simulink model "NucleoTesterScreen"  (R2018a)
settings: Solver=FixedStepAuto  StartTime=0.0  StopTime=10000  FixedStep=0.01  RelTol=1e-3
undefined symbols (not defined in the file): serial
libraries: instrumentlib x6
settings Model: Creator=SIMONE  LastModifiedBy=Salvatore

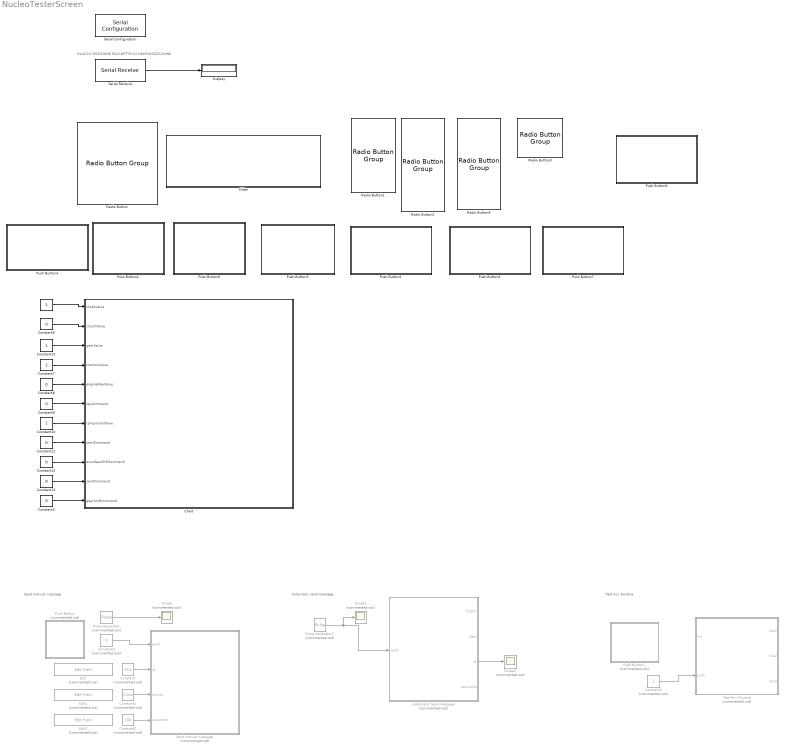
== system NucleoTesterScreen ==
  note: BLOCCO RICEZIONE PACCHETTO DI SINCRONIZZAZIONE
  note: Test Acc Routine
  note: Automatic send message
  note: Send manual message
  " " : Constant  OutDataTypeStr=uint8
  Automatic Send message : Stateflow chart  Commented=on  TreatAsAtomicUnit=on
  Chart : Stateflow chart  TreatAsAtomicUnit=on
  Constant : Constant  Commented=on  Value=513  OutDataTypeStr=uint16
  Constant1 : Constant  Commented=on  Value=21000  OutDataTypeStr=uint16
  Constant10 : Constant  OutDataTypeStr=uint8
  Constant{5,9,11..13} (5 alike) : Constant  Value=0  OutDataTypeStr=uint16
  Constant15 : Constant  OutDataTypeStr=uint8
  Constant2 : Constant  Commented=on  Value=100  OutDataTypeStr=uint16
  Constant3 : Constant  Commented=on  Value=0
  Constant4 : Constant  Commented=on
  Constant6 : Constant  Value=0  OutDataTypeStr=uint8
  Constant7 : Constant  Value=2  OutDataTypeStr=uint8
  Constant8 : Constant  Value=0  OutDataTypeStr=uint8
  Display : Display
  Edit : EditField  Commented=on  WebBlockId=20  LabelPosition=Hide  Alignment=Center
  Edit1 : EditField  Commented=on  WebBlockId=23  LabelPosition=Hide  Alignment=Center
  Edit2 : EditField  Commented=on  WebBlockId=25  LabelPosition=Hide  Alignment=Center
  Pulse Generator : DiscretePulseGenerator  Commented=on  PulseType=Time based  Period=10  PulseWidth=2%  PhaseDelay=1
  Pulse Generator1 : DiscretePulseGenerator  Commented=on  PulseType=Time based  Period=0.2  PulseWidth=25%  PhaseDelay=1
  Push Button : Subsystem  Commented=on  DialogController=hmiCreateDDGDialog  IsWebBlock=on  mask(MWDashboardBlock){webBlockId=12b47424-de0c-4dac-be92-db9266863398, webBlockType=pushbutton, ShowInLibBrwoser=on, ShowInitialText=on, HMISrcModelName=NucleoTesterScreen}
      mask prompts: webBlockId "WebBlock Id"; webBlockType "WebBlock Type"; HMISrcModelName "Source Model"
      mask help: SimulinkHMI:dialogs:PushButtonDialogDesc
      mask Help: helpview([docroot '/mapfiles/simulink.map'], 'hmi_push_button')
      mask Display:
      | model = bdroot(gcb);
      | if strcmp(get_param(model,'BlockDiagramType'), 'library')
      |     image([(matlabroot) '/toolbox/simulink/hmi/icons/PushButton.png']);
      | end
  Push Button1 : Subsystem  Commented=on  DialogController=hmiCreateDDGDialog  IsWebBlock=on  mask(MWDashboardBlock){webBlockId=b87c9129-2ae4-4d53-baa3-891c0a6e6068, webBlockType=pushbutton, ShowInLibBrwoser=on, ShowInitialText=on, HMISrcModelName=NucleoTesterScreen}
      mask prompts: webBlockId "WebBlock Id"; webBlockType "WebBlock Type"; HMISrcModelName "Source Model"
      mask help: SimulinkHMI:dialogs:PushButtonDialogDesc
      mask Help: helpview([docroot '/mapfiles/simulink.map'], 'hmi_push_button')
      mask Display:
      | model = bdroot(gcb);
      | if strcmp(get_param(model,'BlockDiagramType'), 'library')
      |     image([(matlabroot) '/toolbox/simulink/hmi/icons/PushButton.png']);
      | end
  Push Button2 : Subsystem  DialogController=hmiCreateDDGDialog  IsWebBlock=on  mask(MWDashboardBlock){webBlockId=bebfbbc1-03e8-40c0-bb91-fd2048b7631c, webBlockType=pushbutton, ShowInLibBrwoser=on, ShowInitialText=on, HMISrcModelName=NucleoTesterScreen}
      mask prompts: webBlockId "WebBlock Id"; webBlockType "WebBlock Type"; HMISrcModelName "Source Model"
      mask help: SimulinkHMI:dialogs:PushButtonDialogDesc
      mask Help: helpview([docroot '/mapfiles/simulink.map'], 'hmi_push_button')
      mask Display:
      | model = bdroot(gcb);
      | if strcmp(get_param(model,'BlockDiagramType'), 'library')
      |     image([(matlabroot) '/toolbox/simulink/hmi/icons/PushButton.png']);
      | end
  Push Button3 : Subsystem  DialogController=hmiCreateDDGDialog  IsWebBlock=on  mask(MWDashboardBlock){webBlockId=c39a8395-b875-430f-96b1-fe620fcd5c72, webBlockType=pushbutton, ShowInLibBrwoser=on, ShowInitialText=on, HMISrcModelName=NucleoTesterScreen}
      mask prompts: webBlockId "WebBlock Id"; webBlockType "WebBlock Type"; HMISrcModelName "Source Model"
      mask help: SimulinkHMI:dialogs:PushButtonDialogDesc
      mask Help: helpview([docroot '/mapfiles/simulink.map'], 'hmi_push_button')
      mask Display:
      | model = bdroot(gcb);
      | if strcmp(get_param(model,'BlockDiagramType'), 'library')
      |     image([(matlabroot) '/toolbox/simulink/hmi/icons/PushButton.png']);
      | end
  Push Button4 : Subsystem  DialogController=hmiCreateDDGDialog  IsWebBlock=on  mask(MWDashboardBlock){webBlockId=2fda76cb-15c6-45e5-b8fc-bd031a2f9463, webBlockType=pushbutton, ShowInLibBrwoser=on, ShowInitialText=on, HMISrcModelName=NucleoTesterScreen}
      mask prompts: webBlockId "WebBlock Id"; webBlockType "WebBlock Type"; HMISrcModelName "Source Model"
      mask help: SimulinkHMI:dialogs:PushButtonDialogDesc
      mask Help: helpview([docroot '/mapfiles/simulink.map'], 'hmi_push_button')
      mask Display:
      | model = bdroot(gcb);
      | if strcmp(get_param(model,'BlockDiagramType'), 'library')
      |     image([(matlabroot) '/toolbox/simulink/hmi/icons/PushButton.png']);
      | end
  Push Button5 : Subsystem  DialogController=hmiCreateDDGDialog  IsWebBlock=on  mask(MWDashboardBlock){webBlockId=fa35870d-30f4-4e57-b9ad-d2f6e23801ce, webBlockType=pushbutton, ShowInLibBrwoser=on, ShowInitialText=on, HMISrcModelName=NucleoTesterScreen}
      mask prompts: webBlockId "WebBlock Id"; webBlockType "WebBlock Type"; HMISrcModelName "Source Model"
      mask help: SimulinkHMI:dialogs:PushButtonDialogDesc
      mask Help: helpview([docroot '/mapfiles/simulink.map'], 'hmi_push_button')
      mask Display:
      | model = bdroot(gcb);
      | if strcmp(get_param(model,'BlockDiagramType'), 'library')
      |     image([(matlabroot) '/toolbox/simulink/hmi/icons/PushButton.png']);
      | end
  Push Button6 : Subsystem  DialogController=hmiCreateDDGDialog  IsWebBlock=on  mask(MWDashboardBlock){webBlockId=f57953b8-e9ec-4930-bf26-42a61eaad514, webBlockType=pushbutton, ShowInLibBrwoser=on, ShowInitialText=on, HMISrcModelName=NucleoTesterScreen}
      mask prompts: webBlockId "WebBlock Id"; webBlockType "WebBlock Type"; HMISrcModelName "Source Model"
      mask help: SimulinkHMI:dialogs:PushButtonDialogDesc
      mask Help: helpview([docroot '/mapfiles/simulink.map'], 'hmi_push_button')
      mask Display:
      | model = bdroot(gcb);
      | if strcmp(get_param(model,'BlockDiagramType'), 'library')
      |     image([(matlabroot) '/toolbox/simulink/hmi/icons/PushButton.png']);
      | end
  Push Button7 : Subsystem  DialogController=hmiCreateDDGDialog  IsWebBlock=on  mask(MWDashboardBlock){webBlockId=9216e8e9-0fef-4c72-b5a1-64b944c1ca6f, webBlockType=pushbutton, ShowInLibBrwoser=on, ShowInitialText=on, HMISrcModelName=NucleoTesterScreen}
      mask prompts: webBlockId "WebBlock Id"; webBlockType "WebBlock Type"; HMISrcModelName "Source Model"
      mask help: SimulinkHMI:dialogs:PushButtonDialogDesc
      mask Help: helpview([docroot '/mapfiles/simulink.map'], 'hmi_push_button')
      mask Display:
      | model = bdroot(gcb);
      | if strcmp(get_param(model,'BlockDiagramType'), 'library')
      |     image([(matlabroot) '/toolbox/simulink/hmi/icons/PushButton.png']);
      | end
  Push Button8 : Subsystem  DialogController=hmiCreateDDGDialog  IsWebBlock=on  mask(MWDashboardBlock){webBlockId=35ec2f2d-26a3-46c4-8c27-c0d592bab191, webBlockType=pushbutton, ShowInLibBrwoser=on, ShowInitialText=on, HMISrcModelName=NucleoTesterScreen}
      mask prompts: webBlockId "WebBlock Id"; webBlockType "WebBlock Type"; HMISrcModelName "Source Model"
      mask help: SimulinkHMI:dialogs:PushButtonDialogDesc
      mask Help: helpview([docroot '/mapfiles/simulink.map'], 'hmi_push_button')
      mask Display:
      | model = bdroot(gcb);
      | if strcmp(get_param(model,'BlockDiagramType'), 'library')
      |     image([(matlabroot) '/toolbox/simulink/hmi/icons/PushButton.png']);
      | end
  Push Button9 : Subsystem  DialogController=hmiCreateDDGDialog  IsWebBlock=on  mask(MWDashboardBlock){webBlockId=fbcfdafe-b282-4dbd-a33a-70d3112159dd, webBlockType=pushbutton, ShowInLibBrwoser=on, ShowInitialText=on, HMISrcModelName=NucleoTesterScreen}
      mask prompts: webBlockId "WebBlock Id"; webBlockType "WebBlock Type"; HMISrcModelName "Source Model"
      mask help: SimulinkHMI:dialogs:PushButtonDialogDesc
      mask Help: helpview([docroot '/mapfiles/simulink.map'], 'hmi_push_button')
      mask Display:
      | model = bdroot(gcb);
      | if strcmp(get_param(model,'BlockDiagramType'), 'library')
      |     image([(matlabroot) '/toolbox/simulink/hmi/icons/PushButton.png']);
      | end
  Radio Button : RadioButtonGroup  WebBlockId=105  SelectedLabel=Skidpad  ButtonGroupName=MODE
      settings: Values={{'Endurance', 'Acceleration', 'Autocross', 'Skidpad', 'Debug'}, [2 3 0 1 4]}
  Radio Button1 : RadioButtonGroup  WebBlockId=124  SelectedLabel=1  ButtonGroupName=GEAR
      settings: Values={{'1', 'N', '2', '3', '4', '5'}, [1 0 2 3 4 5]}
  Radio Button2 : RadioButtonGroup  WebBlockId=128  SelectedLabel=2  ButtonGroupName=TRACTION
      settings: Values={{'0', '1', '2', '3', '4', '5', '6', '7'}, [0 1 2 3 4 5 6 7]}
  Radio Button3 : RadioButtonGroup  WebBlockId=126  SelectedLabel=MAP 2  ButtonGroupName=ENGINE_MAP
      settings: Values={{'MAP 1', 'MAP 2'}, [1 2]}
  Radio Button4 : RadioButtonGroup  WebBlockId=127  SelectedLabel=1  ButtonGroupName=RPM_LIMITER
      settings: Values={{'0', '1', '2', '3', '4', '5', '6', '7'}, [0 1 2 3 4 5 6 7]}
  Scope : Scope  Commented=on
  Scope1 : Scope  Commented=on
  Scope2 : Scope  Commented=on
  Send manual message : Stateflow chart  Commented=on  TreatAsAtomicUnit=on
  Serial Configuration : instrumentlib/Serial Configuration  Priority=-200000  ComPortMenu=<Please select a port...>  ComPort=COM9  ObjConstructor=serial('COM9');  BaudRate=115200  DataBits=8  Parity=none  StopBits=1  FlowControl=none  Timeout=10  ByteOrder=LittleEndian
  Serial Receive : instrumentlib/Serial Receive  ComPortMenu=<Please select a port...>  ComPort=COM9  ObjConstructor=serial('COM9');  Terminator=<none>  DataSize="[1  1]"  DataType=uint8  EnableBlockingMode=on  ActionDataUnavailable=Output last received value  CustomValue=0  SampleTime=0.01
  Slider : Subsystem  DialogController=hmiCreateDDGDialog  IsWebBlock=on  mask(MWDashboardBlock){webBlockId=fe872d36-e610-44f7-a113-dcc518d376f0, webBlockType=slider, ShowInLibBrowser=on, ShowInitialText=on, HMISrcModelName=NucleoTesterScreen}
      mask prompts: webBlockId "WebBlock Id"; webBlockType "WebBlock Type"; HMISrcModelName "Source Model"
      mask help: SimulinkHMI:dialogs:SliderDialogDesc
      mask Help: helpview([docroot '/mapfiles/simulink.map'], 'hmi_slider')
      mask Display:
      | if strcmp(get_param(bdroot(gcb),'BlockDiagramType'), 'library')
      |     image([(matlabroot) '/toolbox/simulink/hmi/icons/Slider.png']);
      | end
  Test Acc Routine : Subsystem  Commented=on
  wires:
  Constant2/1 -> Send manual message/4(secondInt)
  Constant1/1 -> Send manual message/3(firstInt)
  Constant/1 -> Send manual message/2(id)
  Pulse Generator/1 -> Scope/1
  Pulse Generator1/1 -> Scope1/1, Automatic Send message/1(push)
  Automatic Send message/3(id) -> Scope2/1
  Constant3/1 -> Send manual message/1(push)
  Constant4/1 -> Test Acc Routine/2(push)
  Serial Receive/1 -> Display/1
  " "/1 -> Chart/1(modeValue)
  Constant6/1 -> Chart/2(clutchValue)
  Constant15/1 -> Chart/3(gearValue)
  Constant7/1 -> Chart/4(tractionValue)
  Constant8/1 -> Chart/5(engineMapValue)
  Constant9/1 -> Chart/6(keyCommand)
  Constant10/1 -> Chart/7(rpmLimiterValue)
  Constant11/1 -> Chart/8(startCommand)
  Constant12/1 -> Chart/9(autoGearShiftCommand)
  Constant13/1 -> Chart/10(sendCommand)
  Constant5/1 -> Chart/11(gearShiftCommand)

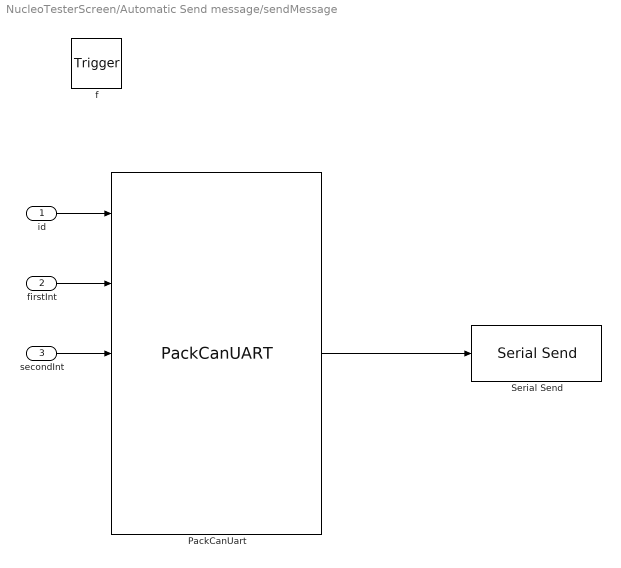
== system NucleoTesterScreen/Automatic Send message/sendMessage ==
  id : Inport  OutDataTypeStr=uint16  PortDimensions=1
  firstInt : Inport  Port=2  OutDataTypeStr=uint16  PortDimensions=1
  secondInt : Inport  Port=3  OutDataTypeStr=uint16  PortDimensions=1
  f : TriggerPort  TriggerType=function-call  VariantControl=(inherit)
      settings: CopyFcn=Stateflow.SLINSF.SimulinkMan.removeBlockPreDeleteFcn  PreDeleteFcn=Stateflow.SLINSF.SimulinkMan.unsafePredeleteFcn
  PackCanUart : S-Function  FunctionName=PackCanUART  SFunctionDeploymentMode=off  EnableBusSupport=off
  Serial Send : instrumentlib/Serial Send  ComPortMenu=<Please select a port...>  ComPort=COM4  ObjConstructor=serial('COM4');  Header=hdr  Terminator=<none>  EnableBlockingMode=on
  wires:
  secondInt/1 -> PackCanUart/3
  firstInt/1 -> PackCanUart/2
  PackCanUart/1 -> Serial Send/1
  id/1 -> PackCanUart/1

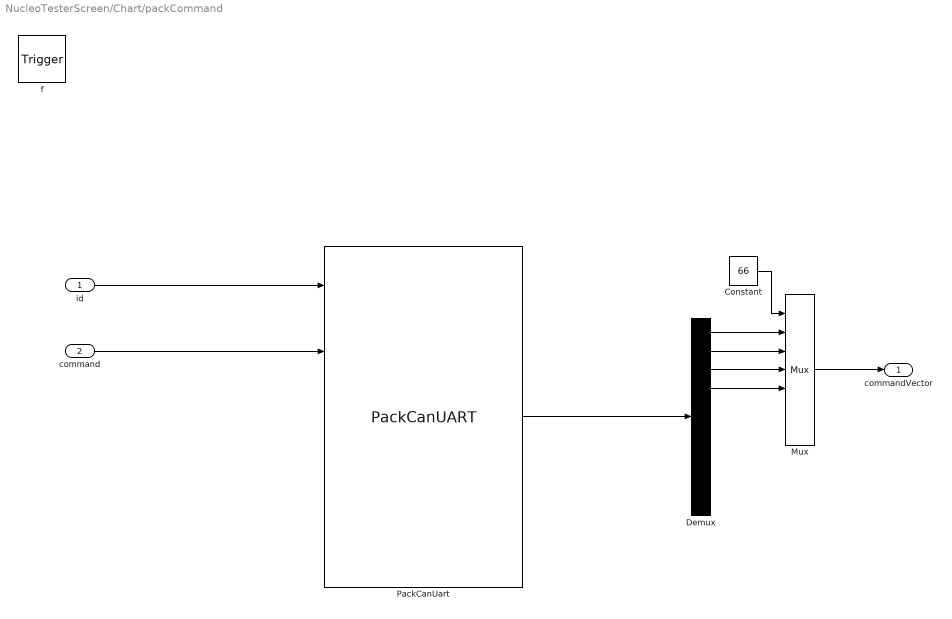
== system NucleoTesterScreen/Chart/packCommand ==
  id : Inport  OutDataTypeStr=uint16  PortDimensions=1
  command : Inport  Port=2  OutDataTypeStr=uint16  PortDimensions=1
  f : TriggerPort  TriggerType=function-call  VariantControl=(inherit)
      settings: CopyFcn=Stateflow.SLINSF.SimulinkMan.removeBlockPreDeleteFcn  PreDeleteFcn=Stateflow.SLINSF.SimulinkMan.unsafePredeleteFcn
  Constant : Constant  Value=66  OutDataTypeStr=uint8
  Demux : Demux  Outputs=10
  Mux : Mux  Inputs=7
  PackCanUart : S-Function  FunctionName=PackCanUART  SFunctionDeploymentMode=off  EnableBusSupport=off
  commandVector : Outport  PortDimensions=[1 7]
  wires:
  id/1 -> PackCanUart/1
  command/1 -> PackCanUart/2
  PackCanUart/1 -> Demux/1
  Mux/1 -> commandVector/1
  Demux/1 -> Mux/2
  Demux/2 -> Mux/3
  Demux/3 -> Mux/4
  Demux/4 -> Mux/5
  Constant/1 -> Mux/1

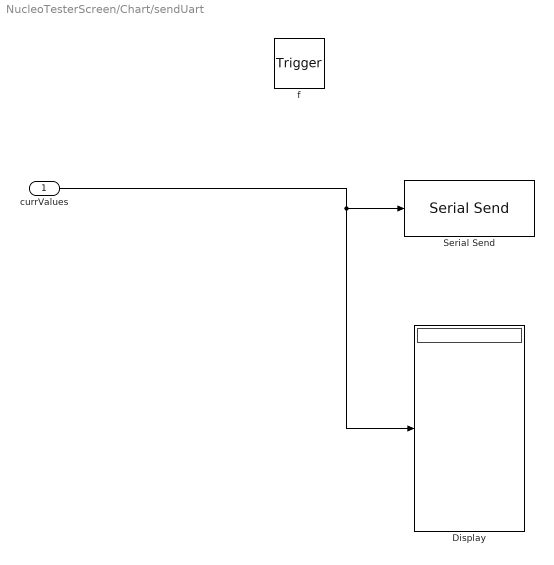
== system NucleoTesterScreen/Chart/sendUart ==
  currValues : Inport  OutDataTypeStr=uint8  PortDimensions=[1,7]
  f : TriggerPort  TriggerType=function-call  VariantControl=(inherit)
      settings: CopyFcn=Stateflow.SLINSF.SimulinkMan.removeBlockPreDeleteFcn  PreDeleteFcn=Stateflow.SLINSF.SimulinkMan.unsafePredeleteFcn
  Display : Display
  Serial Send : instrumentlib/Serial Send  ComPortMenu=COM9  ComPort=COM9  ObjConstructor=serial('COM9');  Terminator=<none>  EnableBlockingMode=on
  wires:
  currValues/1 -> Display/1, Serial Send/1

== system NucleoTesterScreen/Push Button ==

== system NucleoTesterScreen/Push Button1 ==

== system NucleoTesterScreen/Push Button2 ==

== system NucleoTesterScreen/Push Button3 ==

== system NucleoTesterScreen/Push Button4 ==

== system NucleoTesterScreen/Push Button5 ==

== system NucleoTesterScreen/Push Button6 ==

== system NucleoTesterScreen/Push Button7 ==

== system NucleoTesterScreen/Push Button8 ==

== system NucleoTesterScreen/Push Button9 ==

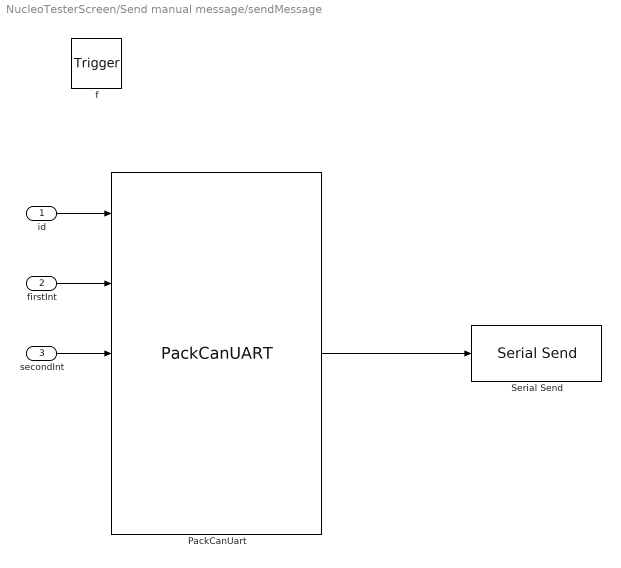
== system NucleoTesterScreen/Send manual message/sendMessage ==
  id : Inport  OutDataTypeStr=uint16  PortDimensions=1
  firstInt : Inport  Port=2  OutDataTypeStr=uint16  PortDimensions=1
  secondInt : Inport  Port=3  OutDataTypeStr=uint16  PortDimensions=1
  f : TriggerPort  TriggerType=function-call  VariantControl=(inherit)
      settings: CopyFcn=Stateflow.SLINSF.SimulinkMan.removeBlockPreDeleteFcn  PreDeleteFcn=Stateflow.SLINSF.SimulinkMan.unsafePredeleteFcn
  PackCanUart : S-Function  FunctionName=PackCanUART  SFunctionDeploymentMode=off  EnableBusSupport=off
  Serial Send : instrumentlib/Serial Send  ComPortMenu=<Please select a port...>  ComPort=COM4  ObjConstructor=serial('COM4');  Header=hdr  Terminator=<none>  EnableBlockingMode=on
  wires:
  secondInt/1 -> PackCanUart/3
  firstInt/1 -> PackCanUart/2
  PackCanUart/1 -> Serial Send/1
  id/1 -> PackCanUart/1

== system NucleoTesterScreen/Slider ==

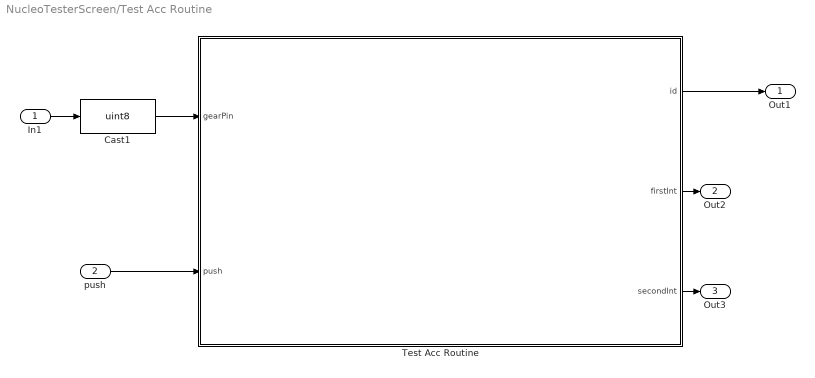
== system NucleoTesterScreen/Test Acc Routine ==
  In1 : Inport
  push : Inport  Port=2
  Cast1 : DataTypeConversion  OutDataTypeStr=uint8
  Test Acc Routine : Stateflow chart  TreatAsAtomicUnit=on  SystemSampleTime=0.05
  Out1 : Outport
  Out2 : Outport  Port=2
  Out3 : Outport  Port=3
  wires:
  In1/1 -> Cast1/1
  Test Acc Routine/1(id) -> Out1/1
  Cast1/1 -> Test Acc Routine/1(gearPin)
  Test Acc Routine/3(secondInt) -> Out3/1
  Test Acc Routine/2(firstInt) -> Out2/1
  push/1 -> Test Acc Routine/2(push)

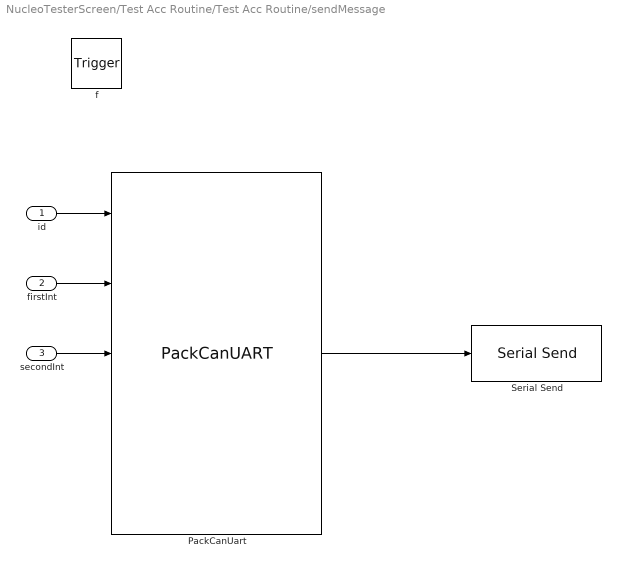
== system NucleoTesterScreen/Test Acc Routine/Test Acc Routine/sendMessage ==
  id : Inport  OutDataTypeStr=uint16  PortDimensions=1
  firstInt : Inport  Port=2  OutDataTypeStr=uint16  PortDimensions=1
  secondInt : Inport  Port=3  OutDataTypeStr=uint16  PortDimensions=1
  f : TriggerPort  TriggerType=function-call  VariantControl=(inherit)
      settings: CopyFcn=Stateflow.SLINSF.SimulinkMan.removeBlockPreDeleteFcn  PreDeleteFcn=Stateflow.SLINSF.SimulinkMan.unsafePredeleteFcn
  PackCanUart : S-Function  FunctionName=PackCanUART  SFunctionDeploymentMode=off  EnableBusSupport=off
  Serial Send : instrumentlib/Serial Send  ComPortMenu=<Please select a port...>  ComPort=COM4  ObjConstructor=serial('COM4');  Header=hdr  Terminator=<none>  EnableBlockingMode=on
  wires:
  secondInt/1 -> PackCanUart/3
  firstInt/1 -> PackCanUart/2
  PackCanUart/1 -> Serial Send/1
  id/1 -> PackCanUart/1

== stateflow chart NucleoTesterScreen/Send manual message ==
  state sendMessage(id,firstInt,secondInt) [function]
  state No_push
  state Push
    entry:
    sendMessage(id, firstInt, secondInt);
  (default) -> No_push
  No_push -> Push : [push==1]
  Push -> No_push : [push==0]
  data: id function_input uint16 size=1; firstInt function_input uint16 size=1; secondInt function_input uint16 size=1; push input; id input uint16; firstInt input uint16; secondInt input uint16

== stateflow chart NucleoTesterScreen/Automatic Send message ==
  state sendMessage(id,firstInt,secondInt) [function]
  state Add [commented out]
    entry:
    %firstInt = 512;
    firstInt=firstInt+256
    sendMessage(id, firstInt, secondInt);
    data = firstInt/256;
  state Subtract [commented out]
    entry:
    %firstInt = 1024;
    firstInt=firstInt+256
    sendMessage(id, firstInt, secondInt);
    data = firstInt/256;
  state setClutch
    entry:
    id = 513;
    firstInt = 65535;
    sendMessage(id, firstInt, secondInt);
  state aacCom
    entry:
    id = 514;
    firstInt = 1;
    sendMessage(id, firstInt, secondInt);
  state GearUpdate
    entry:
    id = 773;
    firstInt=1;
    secondInt = 1000;
    sendMessage(id, firstInt, secondInt);
  state ChangeGear
    entry:
    id = 512;
    firstInt = 400;
    sendMessage(id, firstInt, secondInt);
  state changeMode
    entry:
    id = 1000;
    firstInt = 3;
    sendMessage(id, firstInt, secondInt);
  state aacCom1
    entry:
    id = 514;
    firstInt = 0;
    sendMessage(id, firstInt, secondInt);
  (default) -> Add [commented out]
  Add -> Subtract [commented out] : [data<100]
  Subtract -> Add [commented out] : [data<100]
  (default) -> GearUpdate
  GearUpdate -> setClutch : [push ==1]
  setClutch -> aacCom : [push ==1]
  aacCom -> changeMode : [push ==1]
  changeMode -> aacCom1 : [push ==1]
  aacCom1 -> ChangeGear : [push ==1]
  data: id function_input uint16 size=1; firstInt function_input uint16 size=1; secondInt function_input uint16 size=1; push input; firstInt output uint16 =uint16(0); data output uint16 =uint16(0); id output uint16 =uint16(0); secondInt output uint16 =uint16(0)

== stateflow chart NucleoTesterScreen/Chart ==
  state sendUart(currValues) [function]
  state IDLE
    entry, during: checkCommand;
  state wait
    entry: waitFlag = 0;
  state checkCommand [function]
    (default) -> (junction 34)
    (junction 34) -> (junction 36) [order 1] : [gearShiftCommand > 0]
    (junction 34) -> (junction 40) [order 2]
    (junction 36) -> (junction 110) : {currVector = packCommand(uint16(512), gearShiftCommand);
        | sendUart(currVector);}
    (junction 110) -> (junction 114)
    (junction 114) -> (junction 118)
    (junction 40) -> (junction 42) [order 1] : [startCommand == 1]
    (junction 42) -> (junction 116)
    (junction 40) -> (junction 44) [order 2]
    (junction 44) -> (junction 59) [order 1] : [sendCommand == 1]
    (junction 44) -> (junction 46) [order 2]
    (junction 59) -> (junction 82) : {currValues = [uint8(65), gearValue, clutchValue, modeValue, engineMapValue, tractionValue, rpmLimiterValue];
        | sendUart(currValues);
        | }
    (junction 82) -> (junction 118)
    (junction 118) -> (junction 130) : {waitFlag = 1}
    (junction 46) -> (junction 63) [order 1] : [autoGearShiftCommand == 1]
    (junction 63) -> (junction 120)
    (junction 46) -> (junction 65) [order 2]
    (junction 65) -> (junction 67) [order 1] : [keyCommand == 1]
    (junction 67) -> (junction 121)
    (junction 65) -> (junction 69) [order 2]
  state commandVector = packCommand(id,command) [function]
  (default) -> IDLE
  IDLE -> wait : [waitFlag ==1]
  wait -> IDLE : [sendCommand == 0 && gearShiftCommand == 0]
  data: currValues function_input uint8 size=[1,7]; id function_input uint16 size=1; command function_input uint16 size=1; commandVector function_output size=[1 7]; modeValue input; clutchValue input; gearValue input; tractionValue input; engineMapValue input; keyCommand input; rpmLimiterValue input; startCommand input; autoGearShiftCommand input; sendCommand input; currValues local uint8 size=[1 7]; currCommand local uint8 size=[1 7]; gearShiftCommand input; waitFlag local =0

== stateflow chart NucleoTesterScreen/Test Acc Routine/Test Acc Routine ==
  state Routine [parallel]
    settings: executionOrder=1
    state Wait
    state updateData [function]
      (default) -> (junction 20)
      (junction 20) -> (junction 24) [order 1] : [gearPin == 0 && lastGearPin == 1]
      (junction 20) -> (junction 22) [order 2]
      (junction 24) -> (junction 26) : { currGear = currGear + 1;}
      (junction 26) -> (junction 39)
      (junction 39) -> (junction 43)
      (junction 22) -> (junction 28) [order 1] : [gearPin == 1]
      (junction 22) -> (junction 30) [order 2] : {rpm = rpm + 150; wheelSpeed = wheelSpeed + 5;}
      (junction 28) -> (junction 33) : {rpm = 0; wheelSpeed = 0;}
      (junction 30) -> (junction 33) [order 1] : [message == 0]
      (junction 30) -> (junction 37) [order 2] : {message = 0; id = 774; firstInt = wheelSpeed;}
      (junction 33) -> (junction 35) : {message =1; id = 773; firstInt = currGear; secondInt = rpm;}
      (junction 37) -> (junction 35)
      (junction 35) -> (junction 43)
      (junction 43) -> (junction 46) : {lastGearPin = gearPin;}
    state InsertGear
      entry:
      id = uint16(512);
      firstInt = uint16(400);
      sendMessage(id,firstInt,secondInt)
      during:
      checkGear;
    state Ready
      id = uint16(514);
      firstInt = uint16(2);
      sendMessage(id,firstInt,secondInt)
    state EnterAcceleration
      id = uint16(1000);
      firstInt = uint16(3);
      sendMessage(id,firstInt,secondInt)
    state ActivateAac
      entry:
      id = uint16(514);
      firstInt = uint16(1);
      sendMessage(id,firstInt,secondInt)
    state DajeDeGas
      entry:
      id = uint16(0);
      rpm = uint16(0);
      wheelSpeed = uint16(0);
      during:
      updateData;
      sendMessage(id,firstInt,secondInt)
    state checkGear [function]
      (default) -> (junction 55)
      (junction 55) -> (junction 57) [order 1] : [gearPin == 0 && lastGearPin ==1]
      (junction 55) -> (junction 61) [order 2]
      (junction 57) -> (junction 59) : {currGear = currGear + 1;}
      (junction 59) -> (junction 64)
      (junction 61) -> (junction 64)
      (junction 64) -> (junction 67) : {lastGearPin = gearPin}
    state EXIT
      entry:
      id = uint16(513);
      firstInt = bitshift(uint16(100), 8);
    (default) -> Wait
    Wait -> EnterAcceleration : [push==1]
    InsertGear -> Ready : [currGear ==1 && push==1]
    EnterAcceleration -> ActivateAac : [push==1]
    ActivateAac -> InsertGear : [push==1]
    Ready -> DajeDeGas
  state sendMessage(id,firstInt,secondInt) [function]
  data: id function_input uint16 size=1; firstInt function_input uint16 size=1; secondInt function_input uint16 size=1; id output uint16 =uint16(0); firstInt output uint16 =uint16(0); secondInt output uint16 =uint16(0);; counter local; gearPin input uint8; lastGearPin local uint8 =uint8(0); message local =0; rpm local uint16; wheelSpeed local uint16; currGear local uint16 =uint16(0);; count local; push input
